simulink model "c2"  (R2017a)
settings: Solver=VariableStepAuto  StartTime=0.0  StopTime=1.0  RelTol=1e-3
settings Model: Creator=wuyuche3  LastModifiedBy=wuyuche3

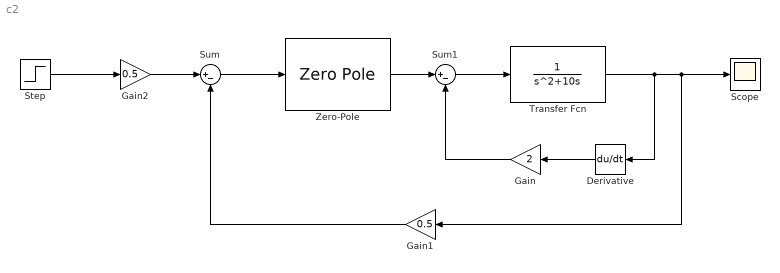
== system c2 ==
  Derivative : Derivative  CoefficientInTFapproximation=0
  Gain : Gain  Gain=2
  Gain1 : Gain  Gain=0.5
  Gain2 : Gain  Gain=0.5
  Scope : Scope
  Step : Step  Time=0  SampleTime=0
  Sum : Sum  Inputs=|+-
  Sum1 : Sum  Inputs=|+-
  Transfer Fcn : TransferFcn  Denominator=[1 10 0]
  Zero-Pole : ZeroPole  Zeros=[-3]  Poles=[-10]  Gain=[1200]
  wires:
  Derivative/1 -> Gain/1
  Gain2/1 -> Sum/1
  Gain1/1 -> Sum/2
  Sum/1 -> Zero-Pole/1
  Zero-Pole/1 -> Sum1/1
  Gain/1 -> Sum1/2
  Sum1/1 -> Transfer Fcn/1
  Transfer Fcn/1 -> Scope/1, Gain1/1, Derivative/1
  Step/1 -> Gain2/1
